simulink model "DC_motor_model"  (R2020a)
settings: Solver=ode45  StartTime=0.0  StopTime=0.2  RelTol=1e-3
undefined symbols (not defined in the file or in its folder): b, J, Kd, Ke, Ki, Kp, Kt, L, R
settings Model: DataDictionary=motor_parameters_dd.sldd  Creator=Viraj  LastModifiedBy=Viraj

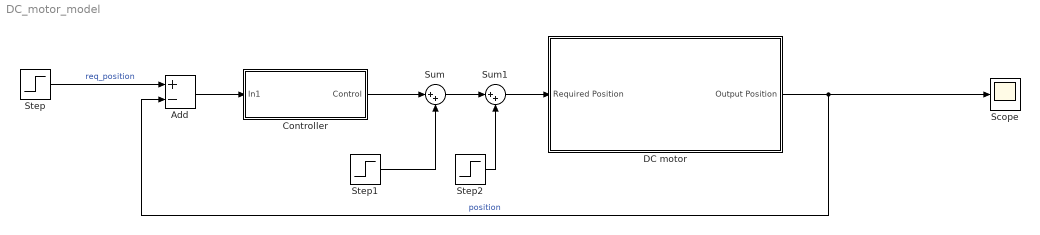
== system DC_motor_model ==
  Add : Sum  Inputs=+-
  Controller : Subsystem
  DC motor : Subsystem
  Scope : Scope
  Step : Step  Time=0  SampleTime=0
  Step1 : Step  Time=0.1  SampleTime=0
  Step2 : Step  Time=0.12  After=-1  SampleTime=0
  Sum : Sum  Inputs=|++
  Sum1 : Sum  Inputs=|++
  wires:
  DC motor/1(Output Position) -> Scope/1, Add/2  "position"
  Step/1 -> Add/1  "req_position"
  Add/1 -> Controller/1(In1)
  Step1/1 -> Sum/2
  Controller/1(Control) -> Sum/1
  Sum/1 -> Sum1/1
  Sum1/1 -> DC motor/1(Required Position)
  Step2/1 -> Sum1/2

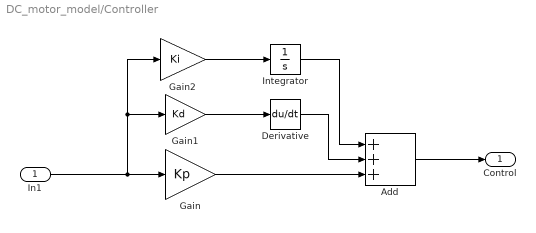
== system DC_motor_model/Controller ==
  In1 : Inport
  Add : Sum  Inputs=+++
  Derivative : Derivative
  Gain : Gain  Gain=Kp
  Gain1 : Gain  Gain=Kd
  Gain2 : Gain  Gain=Ki
  Integrator : Integrator
  Control : Outport
  wires:
  In1/1 -> Gain2/1, Gain1/1, Gain/1
  Gain2/1 -> Integrator/1
  Gain1/1 -> Derivative/1
  Gain/1 -> Add/3
  Derivative/1 -> Add/2
  Integrator/1 -> Add/1
  Add/1 -> Control/1

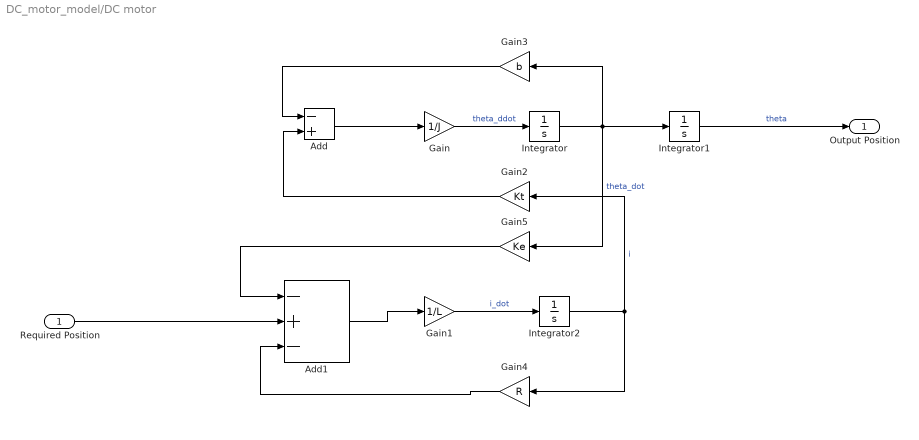
== system DC_motor_model/DC motor ==
  Required Position : Inport
  Add : Sum  Inputs=-+
  Add1 : Sum  Inputs=-+-
  Gain : Gain  Gain=1/J
  Gain1 : Gain  Gain=1/L
  Gain2 : Gain  Gain=Kt
  Gain3 : Gain  Gain=b
  Gain4 : Gain  Gain=R
  Gain5 : Gain  Gain=Ke
  Integrator : Integrator
  Integrator1 : Integrator
  Integrator2 : Integrator
  Output Position : Outport
  wires:
  Integrator2/1 -> Gain2/1, Gain4/1  "i"
  Gain/1 -> Integrator/1  "theta_ddot"
  Required Position/1 -> Add1/2
  Integrator/1 -> Gain3/1, Integrator1/1, Gain5/1  "theta_dot"
  Add1/1 -> Gain1/1
  Add/1 -> Gain/1
  Gain2/1 -> Add/2
  Gain1/1 -> Integrator2/1  "i_dot"
  Integrator1/1 -> Output Position/1  "theta"
  Gain4/1 -> Add1/3
  Gain3/1 -> Add/1
  Gain5/1 -> Add1/1
